simulink subsystem "LQR"  (R2025b)
settings: Solver=VariableStepAuto  StartTime=0.0  StopTime=10.0  RelTol=1e-3
undefined symbols (not defined in the file or in its folder): K_matrix, x1SP, x2SP, x3SP
settings Model: Creator=janek  LastModifiedBy=janek

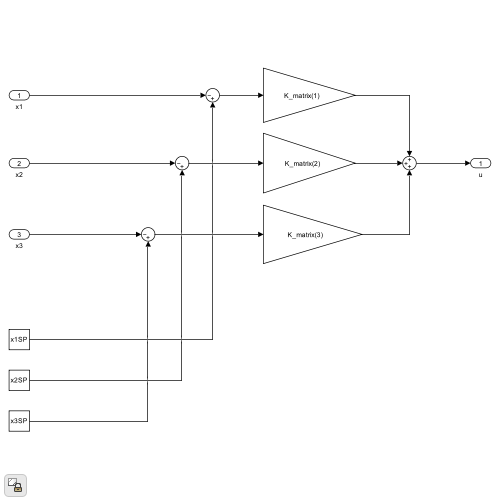
[thumbnail: Simulink's stored preview of the top-level diagram]
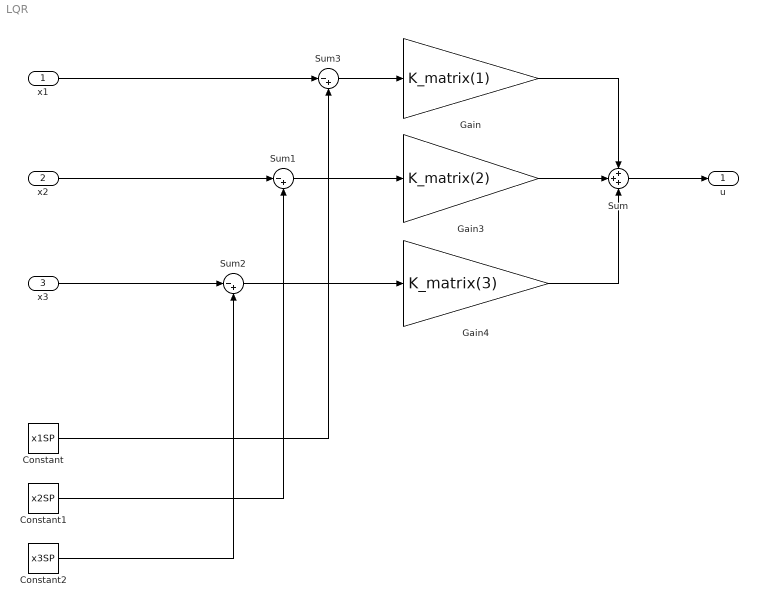
== system LQR ==
  x1 : Inport
  x2 : Inport  Port=2
  x3 : Inport  Port=3
  Constant : Constant  Value=x1SP
  Constant1 : Constant  Value=x2SP
  Constant2 : Constant  Value=x3SP
  Gain : Gain  Gain=K_matrix(1)
  Gain3 : Gain  Gain=K_matrix(2)
  Gain4 : Gain  Gain=K_matrix(3)
  Sum : Sum  Inputs=+++
  Sum1 : Sum  Inputs=|-+
  Sum2 : Sum  Inputs=|-+
  Sum3 : Sum  Inputs=|-+
  u : Outport
  wires:
  x1/1 -> Sum3/1
  x2/1 -> Sum1/1
  Sum3/1 -> Gain/1
  Sum1/1 -> Gain3/1
  Sum2/1 -> Gain4/1
  Sum/1 -> u/1
  Constant/1 -> Sum3/2
  Constant1/1 -> Sum1/2
  Constant2/1 -> Sum2/2
  x3/1 -> Sum2/1
  Gain4/1 -> Sum/3
  Gain/1 -> Sum/1
  Gain3/1 -> Sum/2
